simulink library "libAxisTransformations"  (R2024b)
settings: Solver=ode45  StartTime=0.0  StopTime=10.0  RelTol=1e-3  EnableMultiTasking=on
libraries: libMathOperations x14, starslibAxisTransformations x13, $bdroot x6, starslibMathOperations x2
settings Model: Creator=eheim  LastModifiedBy=gryph
settings SolverCC: AlgebraicLoopSolver=TrustRegion
settings DataIOCC: LimitDataPoints=on  SaveFormat=Array  SignalLoggingSaveFormat=ModelDataLogs  ReturnWorkspaceOutputs=off
settings OptimizationCC: ReuseModelBlockBuffer=off  ExpressionDepthLimit=2147483647  LifeSpan=inf
settings DebuggingCC: UnderspecifiedInitializationDetection=Classic  MergeDetectMultiDrivingBlocksExec=none  SolverPrmCheckMsg=warning  FcnCallInpInsideContextMsg=warning  UnconnectedInputMsg=warning  UnconnectedOutputMsg=warning  UnconnectedLineMsg=warning  StateNameClashWarn=warning  SFUnexpectedBacktrackingDiag=warning  SFNoUnconditionalDefaultTransitionDiag=warning  SFExecutionAtInitializationDiag=none  ArithmeticOperatorsInVariantConditions=warning
settings HardwareCC: ProdBitPerPointer=32  ProdBitPerSizeT=32  ProdBitPerPtrDiffT=32  ProdLargestAtomicFloat=None  ProdIntDivRoundTo=Undefined  ProdEndianess=Unspecified  ProdWordSize=32  ProdHWDeviceType=32-bit Generic
settings ModelReferenceCC: EnableRefExpFcnMdlSchedulingChecks=on  PropagateSignalLabelsOutOfModel=off
settings SFSimCC: SimUseLocalCustomCode=off  CustomCodeUndefinedFunction=UseInterfaceOnly
settings RTWCC: RTWUseLocalCustomCode=off  GPUComputeCapability=3.5  DLArmComputeVersion=19.05
settings CodeAppCC: StateflowObjectComments=on
settings GRTTargetCC: TargetLangStandard=C89/C90 (ANSI)  CombineOutputUpdateFcns=off  GRTInterface=on
settings ConfigComp: CovMetricSettings=dw  CovSaveCumulativeToWorkspaceVar=on  CovSaveSingleToWorkspaceVar=on  CovExternalEMLEnable=off  CovSFcnEnable=off

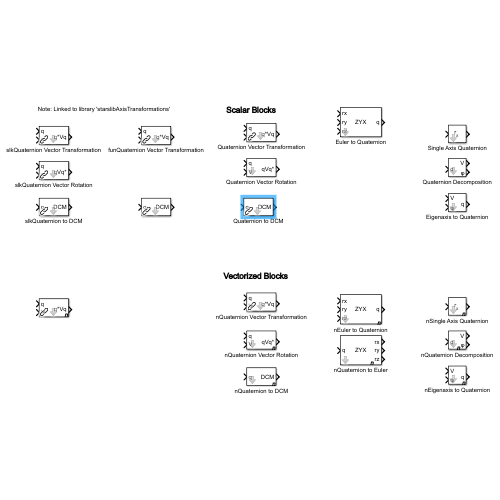
[thumbnail: Simulink's stored preview of the top-level diagram]
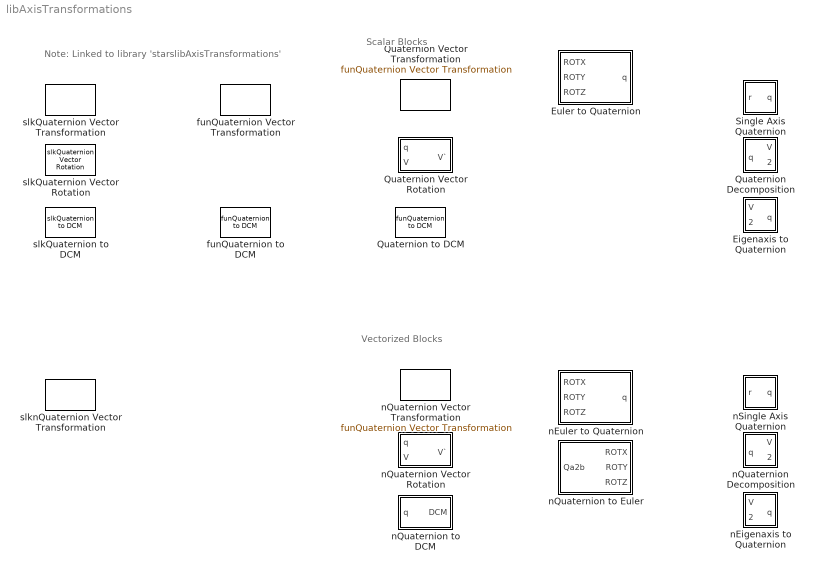
== system libAxisTransformations ==
  note: Note: Linked to library 'starslibAxisTransformations'
  note: Vectorized Blocks
  note: Scalar Blocks
  Eigenaxis to Quaternion : Subsystem  mask(Eigenaxis to Quaternion){n=0}
      mask prompts: n "Hidden variable"
      mask help: Computes quaternion from axis of rotation and angle of rotation.
      mask Display:
      | port_label('input',1,'V')
      | port_label('input',2,'\phi','texmode','on')
      | port_label('output',1,'q')
  Euler to Quaternion : Subsystem  mask(Euler to Quaternion){RotOrd=ZYX, n=0}
      mask prompts: RotOrd "Rotation Order"; n "Hidden variable"
      mask help:
      | Converts multiple Euler angle sets of
      | specified rotation order into quaternions.
      | Quat(:,K) corresponds to ROTX(1,K), ROTY(1,K),
      | and ROTZ(1,K) applied in the specified
      | order (e.g. XYZ,ZYX,...)to ultimately move from one
      | reference frame to another. ROTX, ROTY, and ROTZ
      | are inputed as row vectors with radians units.
      mask init:
      | if RotOrd==1,
      |     irt1=3;irt2=2;irt3=1;RotOrdD='ZYX';
      | elseif RotOrd==2,
      |     irt1=1;irt2=3;irt3=2;RotOrdD='XZY';
      | elseif RotOrd==3,
      |     irt1=2;irt2=1;irt3=3;RotOrdD='YXZ';
      | elseif RotOrd==4,
      |     irt1=3;irt2=1;irt3=2;RotOrdD='ZXY';    
      | elseif RotOrd==5,
      |     irt1=2;irt2=3;irt3=1;RotOrdD='YZX';    
      | elseif RotOrd==6,
      |     irt1=1;irt2=2;irt3=3;RotOrdD='XYZ';
      | end;
      mask TypeOptions RotOrd: ZYX | XZY | YXZ | ZXY | YZX | XYZ
      mask Display:
      | port_label('output',1,'q')
      | port_label('input',1,'rx')
      | port_label('input',2,'ry')
      | port_label('input',3,'rz')
      | disp(RotOrdD)
  Quaternion Decomposition : Subsystem  mask(Quaternion Decomposition){n=0}
      mask prompts: n "Hidden variable"
      mask help: Computes axis of rotation and angle of rotation of quaternion.
      mask Display:
      | port_label('input',1,'q')
      | port_label('output',1,'V')
      | port_label('output',2,'\phi','texmode','on')
  Quaternion Vector Rotation : Subsystem  mask(Quaternion Vector Rotation){n=0}
      mask prompts: n "Hidden variable"
      mask help: Produces quaternion for rotating a vector within a frame.
      mask Display:
      | port_label('input',1,'q')
      | port_label('input',2,'V')
      | port_label('output',1,'qVq*')
  Quaternion Vector Transformation : starslibAxisTransformations/funQuaternion Vector Transformation  n=0
  Quaternion to DCM : starslibAxisTransformations/funQuaternion to DCM  n=0
  Single Axis Quaternion : Subsystem  mask(Quaternion Single Axis Rotation (1-D)){RotAxis=x, n=0}
      mask prompts: RotAxis "Rotation Axis"; n "Hidden variable"
      mask help: Returns quaternion representing rotation of input angle about a selected axis. Input angle must be in radians.
      mask init:
      | switch RotAxis
      |     case 1
      |         A = [1;0;0];
      |         str = 'r_x';
      |     case 2
      |         A = [0;1;0];
      |         str = 'r_y';
      |     case 3
      |         A = [0;0;1];
      |         str = 'r_z';
      | end
      mask TypeOptions RotAxis: x | y | z
      mask Display: text(0.5,0.6,str,'texmode', 'on','HorizontalAlignment','Center','VerticalAlignment','Middle')
  funQuaternion Vector Transformation : starslibAxisTransformations/funQuaternion Vector Transformation  n=0
  funQuaternion to DCM : starslibAxisTransformations/funQuaternion to DCM  n=0
  nEigenaxis to Quaternion : Subsystem  mask(nEigenaxis to Quaternion){n=1}
      mask prompts: n "Number of Quaternions"
      mask help: Computes quaternion from axis of rotation and angle of rotation.
      mask Display:
      | port_label('input',1,'V')
      | port_label('input',2,'\phi','texmode','on')
      | port_label('output',1,'q')
      | text(1,0,'\bf\it{n}','texmode','on','HorizontalAlignment','Right','VerticalAlignment','base')
  nEuler to Quaternion : Subsystem  mask(nEuler to Quaternion){RotOrd=ZYX, n=1}
      mask prompts: RotOrd "Rotation Order"; n "Number of Quaternions"
      mask help:
      | Converts multiple Euler angle sets of
      | specified rotation order into quaternions.
      | Quat(:,K) corresponds to ROTX(1,K), ROTY(1,K),
      | and ROTZ(1,K) applied in the specified
      | order (e.g. XYZ,ZYX,...)to ultimately move from one
      | reference frame to another. ROTX, ROTY, and ROTZ
      | are inputed as row vectors with radians units.
      mask init: same as libAxisTransformations/Euler to Quaternion
      mask TypeOptions RotOrd: ZYX | XZY | YXZ | ZXY | YZX | XYZ
      mask Display:
      | port_label('output',1,'q')
      | port_label('input',1,'rx')
      | port_label('input',2,'ry')
      | port_label('input',3,'rz')
      | disp(RotOrdD)
      | text(1,0,'\bf\it{n}','texmode','on','HorizontalAlignment','Right','VerticalAlignment','base')
  nQuaternion Decomposition : Subsystem  mask(nQuaternion Decomposition){n=1}
      mask prompts: n "Number of Quaternions"
      mask help: Computes axis of rotation and angle of rotation of quaternion.
      mask Display:
      | port_label('input',1,'q')
      | port_label('output',1,'V')
      | port_label('output',2,'\phi','texmode','on')
      | text(0.5,0,'\bf\it{n}','texmode','on','HorizontalAlignment','Left','VerticalAlignment','base')
  nQuaternion Vector Rotation : Subsystem  mask(nQuaternion Vector Rotation){n=1}
      mask prompts: n "Number of Quaternions"
      mask help: Produces quaternion for rotating a vector within a frame.
      mask Display:
      | port_label('input',1,'q')
      | port_label('input',2,'V')
      | port_label('output',1,'qVq*')
      | text(1,0,'\bf\it{n}','texmode','on','HorizontalAlignment','Right','VerticalAlignment','base')
  nQuaternion Vector Transformation : starslibAxisTransformations/funQuaternion Vector Transformation  n=0
  nQuaternion to DCM : Subsystem  mask(nQuaternion to DCM){n=1}
      mask prompts: n "Number of Quaternions"
      mask help:
      | Converts n Quaternions into Direction Cosine Matrices (DCM).
      | The DCM of q(:,k) is reshape(DCM(:,k),3,3).
      mask Display:
      | port_label('input',1,'q')
      | port_label('output',1,'DCM')
      | text(1,0,'\bf\it{n}','texmode','on','HorizontalAlignment','Right','VerticalAlignment','base')
  nQuaternion to Euler : Subsystem  mask(Quaternion to Euler(4xN)){n=1, RotOrd=ZYX}
      mask prompts: n "Number of Quaternions"; RotOrd "Rotation Order"
      mask help:
      | Converts multiple quaternions (cols of input matrix)
      | into Euler angles of specified rotation order
      | (e.g. XYZ,ZYX,...).  Outputs ROTX designate rotation
      | required in x-axis, ROTY is the required rotation in the
      | y axis,and ROTZ is the required rotation in the z axis.
      | All outputs are in radians.
      mask init:
      | U1=eye(3);
      | DirCrx=[2 3; 3 1;1 2];
      | if RotOrd==1,
      |     irt1=3;irt2=2;irt3=1;RotOrdD='ZYX';
      | elseif RotOrd==2,
      |     irt1=1;irt2=3;irt3=2;RotOrdD='XZY';
      | elseif RotOrd==3,
      |     irt1=2;irt2=1;irt3=3;RotOrdD='YXZ';
      | elseif RotOrd==4,
      |     irt1=3;irt2=1;irt3=2;RotOrdD='ZXY';    
      | elseif RotOrd==5,
      |     irt1=2;irt2=3;irt3=1;RotOrdD='YZX';    
      | elseif RotOrd==6,
      |     irt1=1;irt2=2;irt3=3;RotOrdD='XYZ';
      | end;
      mask TypeOptions RotOrd: ZYX | XZY | YXZ | ZXY | YZX | XYZ
      mask Display:
      | port_label('input',1,'q')
      | port_label('output',1,'rx')
      | port_label('output',2,'ry')
      | port_label('output',3,'rz')
      | disp(RotOrdD)
      | text(0.75,0,'\bf\it{n}','texmode','on','HorizontalAlignment','Left','VerticalAlignment','base')
  nSingle Axis Quaternion : Subsystem  mask(nSingle Axis Quaternion){RotAxis=x, n=1}
      mask prompts: RotAxis "Rotation Axis"; n "Number of Angles"
      mask help: Returns quaternion(s) representing rotation(s) of input angle about a selected axis. Input angle must be in radians.
      mask init:
      | switch RotAxis
      |     case 1
      |         A = [1;0;0];
      |         str = 'r_x';
      |     case 2
      |         A = [0;1;0];
      |         str = 'r_y';
      |     case 3
      |         A = [0;0;1];
      |         str = 'r_z';
      | end
      mask TypeOptions RotAxis: x | y | z
      mask Display:
      | text(0.5,0.6,str,'texmode', 'on','HorizontalAlignment','Center','VerticalAlignment','Middle')
      | text(1,0,'\bf\it{n}','texmode','on','HorizontalAlignment','Right','VerticalAlignment','base')
  slkQuaternion Vector Rotation : starslibAxisTransformations/slkQuaternion Vector Rotation  n=0
  slkQuaternion Vector Transformation : starslibAxisTransformations/slkQuaternion Vector Transformation  n=0
  slkQuaternion to DCM : starslibAxisTransformations/slkQuaternion to DCM  n=0
  slknQuaternion Vector Transformation : starslibAxisTransformations/slknQuaternion Vector Transformation  n=1

== system libAxisTransformations/Eigenaxis to Quaternion ==
  V : Inport
  phi : Inport  Port=2
  Gain1 : Gain  Gain=0.5
  Mux : Mux  Inputs=2
  Mux1 : Mux  Inputs=3
  Normalize Vector : libMathOperations/Normalize Vector  dimnorm=rows  n=1
  Product3 : Product  RndMeth=Zero
  Quaternion Normalize : libMathOperations/Quaternion Normalize  n=0
  Trigonometric Function2 : Trigonometry  Operator=sincos
  q : Outport
  wires:
  Normalize Vector/1 -> Product3/1
  Trigonometric Function2/1 -> Mux1/2, Mux1/1, Mux1/3
  Mux1/1 -> Product3/2
  phi/1 -> Gain1/1
  Gain1/1 -> Trigonometric Function2/1
  V/1 -> Normalize Vector/1
  Product3/1 -> Mux/2
  Trigonometric Function2/2 -> Mux/1
  Mux/1 -> Quaternion Normalize/1
  Quaternion Normalize/1 -> q/1

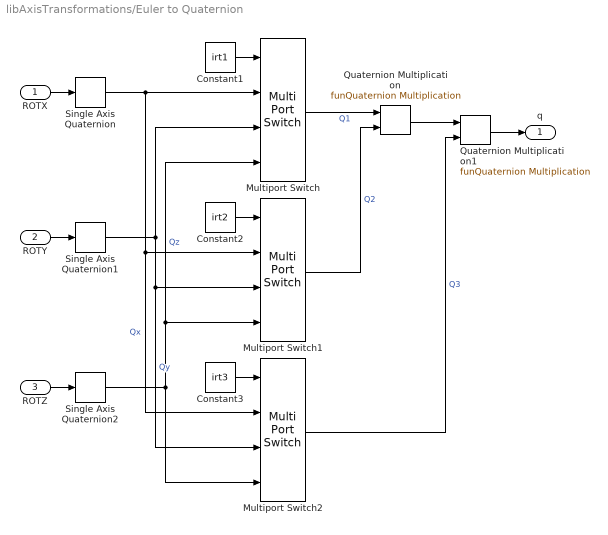
== system libAxisTransformations/Euler to Quaternion ==
  ROTX : Inport
  ROTY : Inport  Port=2
  ROTZ : Inport  Port=3
  Constant1 : Constant  Value=irt1  VectorParams1D=off
  Constant2 : Constant  Value=irt2  VectorParams1D=off
  Constant3 : Constant  Value=irt3  VectorParams1D=off
  Multiport Switch : MultiPortSwitch  SaturateOnIntegerOverflow=off  InputSameDT=off
  Multiport Switch1 : MultiPortSwitch  SaturateOnIntegerOverflow=off  InputSameDT=off
  Multiport Switch2 : MultiPortSwitch  SaturateOnIntegerOverflow=off  InputSameDT=off
  Quaternion Multiplication : starslibMathOperations/funQuaternion Multiplication  n=0
  Quaternion Multiplication1 : starslibMathOperations/funQuaternion Multiplication  n=0
  Single Axis Quaternion : $bdroot/Single Axis Quaternion  RotAxis=x  n=0
  Single Axis Quaternion1 : $bdroot/Single Axis Quaternion  RotAxis=y  n=0
  Single Axis Quaternion2 : $bdroot/Single Axis Quaternion  RotAxis=z  n=0
  q : Outport
  wires:
  Constant1/1 -> Multiport Switch/1
  Constant2/1 -> Multiport Switch1/1
  Constant3/1 -> Multiport Switch2/1
  ROTX/1 -> Single Axis Quaternion/1
  ROTZ/1 -> Single Axis Quaternion2/1
  ROTY/1 -> Single Axis Quaternion1/1
  Single Axis Quaternion/1 -> Multiport Switch/2, Multiport Switch1/2, Multiport Switch2/2  "Qx"
  Single Axis Quaternion1/1 -> Multiport Switch/3, Multiport Switch1/3, Multiport Switch2/3  "Qy"
  Single Axis Quaternion2/1 -> Multiport Switch/4, Multiport Switch1/4, Multiport Switch2/4  "Qz"
  Multiport Switch/1 -> Quaternion Multiplication/1  "Q1"
  Multiport Switch1/1 -> Quaternion Multiplication/2  "Q2"
  Quaternion Multiplication/1 -> Quaternion Multiplication1/1
  Multiport Switch2/1 -> Quaternion Multiplication1/2  "Q3"
  Quaternion Multiplication1/1 -> q/1

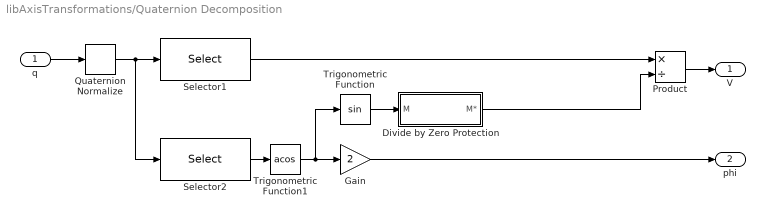
== system libAxisTransformations/Quaternion Decomposition ==
  q : Inport
  Divide by Zero Protection : Subsystem
  Gain : Gain  Gain=2
  Product : Product  Inputs=*/  RndMeth=Zero
  Quaternion Normalize : libMathOperations/Quaternion Normalize  n=0
  Selector1 : Selector  InputPortWidth=4  IndexOptions=Index vector (dialog)  Indices=[2 3 4]  OutputSizes=1
  Selector2 : Selector  InputPortWidth=4  IndexOptions=Index vector (dialog)  Indices=1  OutputSizes=1
  Trigonometric Function : Trigonometry
  Trigonometric Function1 : Trigonometry  Operator=acos
  V : Outport
  phi : Outport  Port=2
  wires:
  Divide by Zero Protection/1(M*) -> Product/2
  Trigonometric Function/1 -> Divide by Zero Protection/1(M)
  Gain/1 -> phi/1
  Trigonometric Function1/1 -> Trigonometric Function/1, Gain/1
  Selector2/1 -> Trigonometric Function1/1
  Selector1/1 -> Product/1
  Quaternion Normalize/1 -> Selector2/1, Selector1/1
  q/1 -> Quaternion Normalize/1
  Product/1 -> V/1

== system libAxisTransformations/Quaternion Vector Rotation ==
  q : Inport
  V : Inport  Port=2
  Quaternion Conjugate : libMathOperations/Quaternion Conjugate  n=0
  Subsystem6 : Subsystem  mask(Quat Mult for two special sets of quaternions){}
      mask help:
      | Quaternion multiplication of two sets of quaternions. First element assumed
      | zero of second Quaternion.  Input only last three elements
      | of second quaternion.
      mask Display:
      | disp('Quat Mult\n q0=0')
      | port_label('input',1,'p')
      | port_label('input',2,'q')
      | port_label('output',1,'p*q')
  Subsystem7 : Subsystem  mask(Quat Mult for two sets of quaternions){}
      mask help:
      | Quaternion multiplication of two sets of quaternions.  Outputs only last
      | three elements of product.
      mask Display:
      | disp('Quat Mult\n 1st Row\nRemoved')
      | port_label('input',1,'p')
      | port_label('input',2,'q')
      | port_label('output',1,'p*q')
  V` : Outport
  wires:
  Subsystem6/1(p * q) -> Subsystem7/1(p)
  q/1 -> Subsystem6/1(p), Quaternion Conjugate/1
  Subsystem7/1(p * q) -> V`/1
  V/1 -> Subsystem6/2(q)
  Quaternion Conjugate/1 -> Subsystem7/2(q)

== system libAxisTransformations/Single Axis Quaternion ==
  r : Inport
  Gain : Gain  Gain=A
  Gain3 : Gain  Gain=.5
  Mux : Mux  Inputs=2
  Trigonometric Function1 : Trigonometry  Operator=cos
  Trigonometric Function2 : Trigonometry
  q : Outport
  wires:
  Gain3/1 -> Trigonometric Function2/1, Trigonometric Function1/1
  Trigonometric Function1/1 -> Mux/1
  Gain/1 -> Mux/2
  Trigonometric Function2/1 -> Gain/1
  r/1 -> Gain3/1
  Mux/1 -> q/1

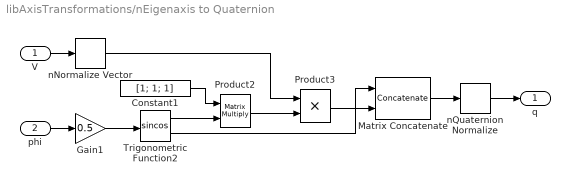
== system libAxisTransformations/nEigenaxis to Quaternion ==
  V : Inport  PortDimensions=[3,n]
  phi : Inport  Port=2  PortDimensions=[1,n]
  Constant1 : Constant  Value=[1; 1; 1]  VectorParams1D=off
  Gain1 : Gain  Gain=0.5
  Matrix Concatenate : Concatenate  Mode=Multidimensional array
  Product2 : Product  Multiplication=Matrix(*)  RndMeth=Zero
  Product3 : Product  RndMeth=Zero
  Trigonometric Function2 : Trigonometry  Operator=sincos
  nNormalize Vector : libMathOperations/nNormalize Vector  dimnorm=rows  n=[3, n]
  nQuaternion Normalize : libMathOperations/nQuaternion Normalize  n=n
  q : Outport  PortDimensions=[4,n]
  wires:
  phi/1 -> Gain1/1
  Gain1/1 -> Trigonometric Function2/1
  Constant1/1 -> Product2/1
  Trigonometric Function2/1 -> Product2/2
  Product2/1 -> Product3/2
  V/1 -> nNormalize Vector/1
  Product3/1 -> Matrix Concatenate/2
  Trigonometric Function2/2 -> Matrix Concatenate/1
  Matrix Concatenate/1 -> nQuaternion Normalize/1
  nQuaternion Normalize/1 -> q/1
  nNormalize Vector/1 -> Product3/1

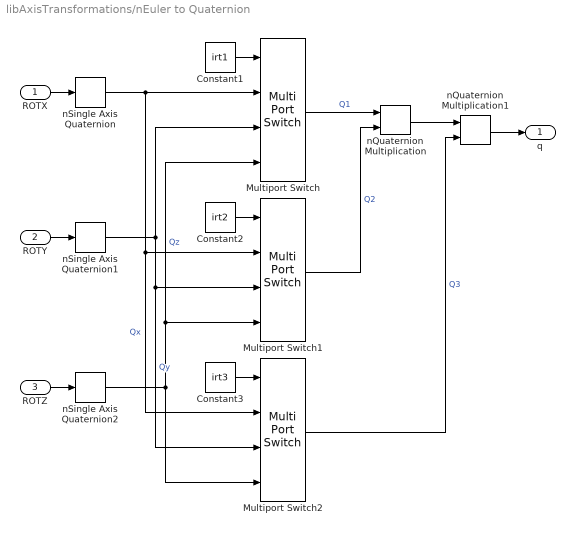
== system libAxisTransformations/nEuler to Quaternion ==
  ROTX : Inport  PortDimensions=[1,n]
  ROTY : Inport  Port=2  PortDimensions=[1,n]
  ROTZ : Inport  Port=3  PortDimensions=[1,n]
  Constant1 : Constant  Value=irt1  VectorParams1D=off
  Constant2 : Constant  Value=irt2  VectorParams1D=off
  Constant3 : Constant  Value=irt3  VectorParams1D=off
  Multiport Switch : MultiPortSwitch  SaturateOnIntegerOverflow=off  InputSameDT=off
  Multiport Switch1 : MultiPortSwitch  SaturateOnIntegerOverflow=off  InputSameDT=off
  Multiport Switch2 : MultiPortSwitch  SaturateOnIntegerOverflow=off  InputSameDT=off
  nQuaternion Multiplication : libMathOperations/nQuaternion Multiplication  n=n
  nQuaternion Multiplication1 : libMathOperations/nQuaternion Multiplication  n=n
  nSingle Axis Quaternion : $bdroot/nSingle Axis Quaternion  RotAxis=x  n=n
  nSingle Axis Quaternion1 : $bdroot/nSingle Axis Quaternion  RotAxis=y  n=n
  nSingle Axis Quaternion2 : $bdroot/nSingle Axis Quaternion  RotAxis=z  n=n
  q : Outport  PortDimensions=[4,n]
  wires:
  Constant1/1 -> Multiport Switch/1
  Constant2/1 -> Multiport Switch1/1
  Constant3/1 -> Multiport Switch2/1
  ROTX/1 -> nSingle Axis Quaternion/1
  ROTZ/1 -> nSingle Axis Quaternion2/1
  ROTY/1 -> nSingle Axis Quaternion1/1
  nSingle Axis Quaternion/1 -> Multiport Switch/2, Multiport Switch1/2, Multiport Switch2/2  "Qx"
  nSingle Axis Quaternion1/1 -> Multiport Switch/3, Multiport Switch1/3, Multiport Switch2/3  "Qy"
  nSingle Axis Quaternion2/1 -> Multiport Switch/4, Multiport Switch1/4, Multiport Switch2/4  "Qz"
  Multiport Switch/1 -> nQuaternion Multiplication/1  "Q1"
  Multiport Switch1/1 -> nQuaternion Multiplication/2  "Q2"
  nQuaternion Multiplication/1 -> nQuaternion Multiplication1/1
  Multiport Switch2/1 -> nQuaternion Multiplication1/2  "Q3"
  nQuaternion Multiplication1/1 -> q/1

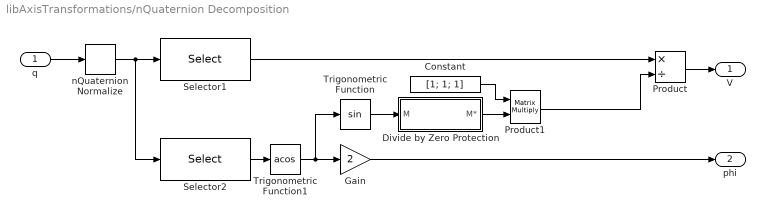
== system libAxisTransformations/nQuaternion Decomposition ==
  q : Inport  PortDimensions=[4,n]
  Constant : Constant  Value=[1; 1; 1]  VectorParams1D=off
  Divide by Zero Protection : Subsystem
  Gain : Gain  Gain=2
  Product : Product  Inputs=*/  RndMeth=Zero
  Product1 : Product  Multiplication=Matrix(*)  RndMeth=Zero
  Selector1 : Selector  NumberOfDimensions=2  InputPortWidth=3  IndexOptions=Index vector (dialog),Select all  Indices=[2 3 4],1  OutputSizes=1,1
  Selector2 : Selector  NumberOfDimensions=2  InputPortWidth=3  IndexOptions=Index vector (dialog),Select all  Indices=1,1  OutputSizes=1,1
  Trigonometric Function : Trigonometry
  Trigonometric Function1 : Trigonometry  Operator=acos
  nQuaternion Normalize : libMathOperations/nQuaternion Normalize  n=n
  V : Outport  PortDimensions=[3,n]
  phi : Outport  Port=2  PortDimensions=[1,n]
  wires:
  Divide by Zero Protection/1(M*) -> Product1/2
  Trigonometric Function/1 -> Divide by Zero Protection/1(M)
  Gain/1 -> phi/1
  Trigonometric Function1/1 -> Trigonometric Function/1, Gain/1
  Selector2/1 -> Trigonometric Function1/1
  Selector1/1 -> Product/1
  nQuaternion Normalize/1 -> Selector2/1, Selector1/1
  q/1 -> nQuaternion Normalize/1
  Product/1 -> V/1
  Product1/1 -> Product/2
  Constant/1 -> Product1/1

== system libAxisTransformations/nQuaternion Vector Rotation ==
  q : Inport  PortDimensions=[4,n]
  V : Inport  Port=2  PortDimensions=[3,n]
  Subsystem6 : Subsystem  mask(Quat Mult for two special sets of quaternions){nQuat=n}
      mask prompts: nQuat "Number of quaternions in input"
      mask help:
      | Quaternion multiplication of two sets of quaternions
      | inputted by 2 (4 x nQuat) matrices. First element assumed
      | zero of second Quaternion.  Input only last three elements
      | of second quaternion.  Used in Qtrans' first quaternion
      | multiplication
      mask Display:
      | disp('n-Quat Mult\n q0=0')
      | port_label('input',1,'p')
      | port_label('input',2,'q')
      | port_label('output',1,'p*q')
  Subsystem7 : Subsystem  mask(Quat Mult for two sets of quaternions){nQuat=n}
      mask prompts: nQuat "Number of quaternions in input"
      mask help:
      | Quaternion multiplication of two sets of quaternions
      | inputted by 2 (4 x nQuat) matrices.  Outputs only last
      | three elements of product.  Used in QTrans' second
      | multiplication
      mask Display:
      | disp('n-Quat Mult\n 1st Row\nRemoved')
      | port_label('input',1,'p')
      | port_label('input',2,'q')
      | port_label('output',1,'p*q')
  nQuaternion Conjugate : libMathOperations/nQuaternion Conjugate  n=n
  V` : Outport  PortDimensions=[3,n]
  wires:
  q/1 -> Subsystem6/1(p), nQuaternion Conjugate/1
  Subsystem6/1(p * q) -> Subsystem7/1(p)
  Subsystem7/1(p * q) -> V`/1
  V/1 -> Subsystem6/2(q)
  nQuaternion Conjugate/1 -> Subsystem7/2(q)

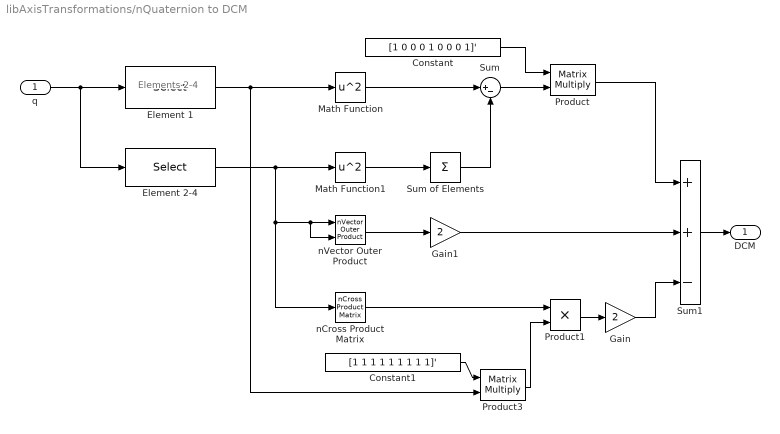
== system libAxisTransformations/nQuaternion to DCM ==
  note: Elements 2-4
  q : Inport  PortDimensions=[4,n]
  Constant : Constant  Value=[1 0 0 0 1 0 0 0 1]'  VectorParams1D=off
  Constant1 : Constant  Value=[1 1 1 1 1 1 1 1 1]'  VectorParams1D=off
  Element 1 : Selector  NumberOfDimensions=2  InputPortWidth=3  IndexOptions=Index vector (dialog),Select all  Indices=[1],1  OutputSizes=1,1
  Element 2-4 : Selector  NumberOfDimensions=2  InputPortWidth=3  IndexOptions=Index vector (dialog),Select all  Indices=[2 3 4],1  OutputSizes=1,1
  Gain : Gain  Gain=2
  Gain1 : Gain  Gain=2
  Math Function : Math  Operator=square  SignedPower=on
  Math Function1 : Math  Operator=square  SignedPower=on
  Product : Product  Multiplication=Matrix(*)  RndMeth=Zero
  Product1 : Product  RndMeth=Zero
  Product3 : Product  Multiplication=Matrix(*)  RndMeth=Zero
  Sum : Sum  Inputs=|+-
  Sum of Elements : Sum  Inputs=+  CollapseMode=Specified dimension
  Sum1 : Sum  Inputs=++-
  nCross Product Matrix : libMathOperations/nCross Product Matrix  n=n
  nVector Outer Product : libMathOperations/nVector Outer Product  n=n
  DCM : Outport  PortDimensions=[9,n]
  wires:
  Gain/1 -> Sum1/3
  Gain1/1 -> Sum1/2
  Product3/1 -> Product1/2
  Constant1/1 -> Product3/1
  nCross Product Matrix/1 -> Product1/1
  Product1/1 -> Gain/1
  Sum1/1 -> DCM/1
  Product/1 -> Sum1/1
  nVector Outer Product/1 -> Gain1/1
  Constant/1 -> Product/1
  Sum/1 -> Product/2
  Sum of Elements/1 -> Sum/2
  Math Function/1 -> Sum/1
  Math Function1/1 -> Sum of Elements/1
  Element 2-4/1 -> nVector Outer Product/1, nVector Outer Product/2, nCross Product Matrix/1, Math Function1/1
  Element 1/1 -> Product3/2, Math Function/1
  q/1 -> Element 1/1, Element 2-4/1

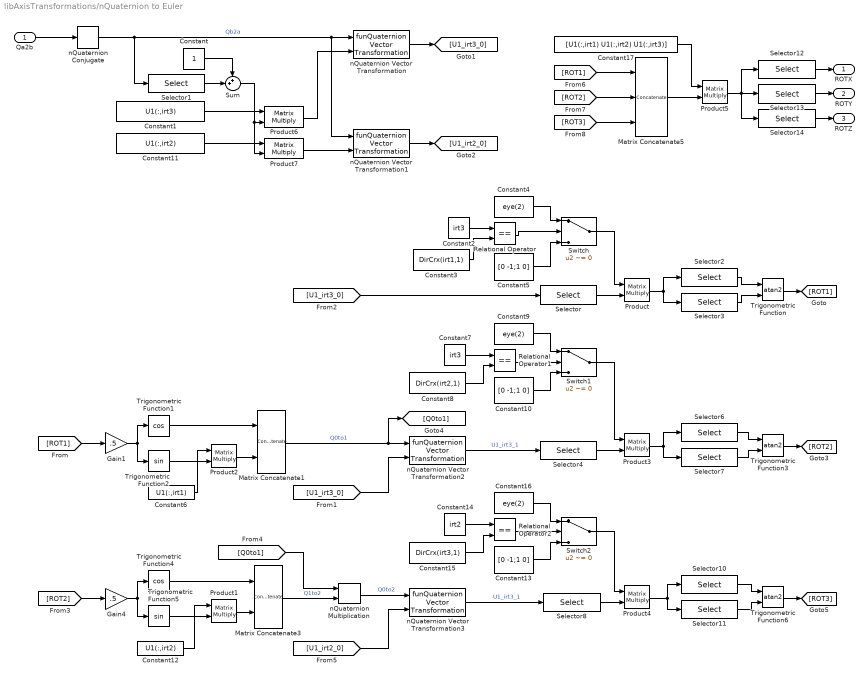
== system libAxisTransformations/nQuaternion to Euler ==
  Qa2b : Inport  PortDimensions=[4,n]
  Constant : Constant
  Constant1 : Constant  Value=U1(:,irt3)  VectorParams1D=off
  Constant10 : Constant  Value=[0 -1;1 0]  VectorParams1D=off
  Constant11 : Constant  Value=U1(:,irt2)  VectorParams1D=off
  Constant12 : Constant  Value=U1(:,irt2)  VectorParams1D=off
  Constant13 : Constant  Value=[0 -1;1 0]  VectorParams1D=off
  Constant14 : Constant  Value=irt2  VectorParams1D=off
  Constant15 : Constant  Value=DirCrx(irt3,1)  VectorParams1D=off
  Constant16 : Constant  Value=eye(2)  VectorParams1D=off
  Constant17 : Constant  Value=[U1(:,irt1) U1(:,irt2) U1(:,irt3)]  VectorParams1D=off
  Constant2 : Constant  Value=irt3  VectorParams1D=off
  Constant3 : Constant  Value=DirCrx(irt1,1)  VectorParams1D=off
  Constant4 : Constant  Value=eye(2)  VectorParams1D=off
  Constant5 : Constant  Value=[0 -1;1 0]  VectorParams1D=off
  Constant6 : Constant  Value=U1(:,irt1)  VectorParams1D=off
  Constant7 : Constant  Value=irt3  VectorParams1D=off
  Constant8 : Constant  Value=DirCrx(irt2,1)  VectorParams1D=off
  Constant9 : Constant  Value=eye(2)  VectorParams1D=off
  Gain1 : Gain  Gain=.5
  Gain4 : Gain  Gain=.5
  Matrix Concatenate1 : Concatenate  Mode=Multidimensional array
  Matrix Concatenate3 : Concatenate  Mode=Multidimensional array
  Matrix Concatenate5 : Concatenate  NumInputs=3  Mode=Multidimensional array
  Product{,1..7} (8 alike) : Product  Multiplication=Matrix(*)  RndMeth=Zero
  Relational Operator : RelationalOperator  Operator===  OutDataTypeStr=boolean  ZeroCross=off  InputSameDT=off
  Relational Operator1 : RelationalOperator  Operator===  OutDataTypeStr=boolean  ZeroCross=off  InputSameDT=off
  Relational Operator2 : RelationalOperator  Operator===  OutDataTypeStr=boolean  ZeroCross=off  InputSameDT=off
  Selector : Selector  NumberOfDimensions=2  InputPortWidth=3  IndexOptions=Index vector (dialog),Select all  Indices=[DirCrx(irt1,2) DirCrx(irt1,1)],1  OutputSizes=1,1
  Selector{1..2,6,10,12} (5 alike) : Selector  NumberOfDimensions=2  InputPortWidth=3  IndexOptions=Index vector (dialog),Select all  Indices=1,1  OutputSizes=1,1
  Selector{3,7,11,13} (4 alike) : Selector  NumberOfDimensions=2  InputPortWidth=3  IndexOptions=Index vector (dialog),Select all  Indices=2,1  OutputSizes=1,1
  Selector14 : Selector  NumberOfDimensions=2  InputPortWidth=3  IndexOptions=Index vector (dialog),Select all  Indices=3,1  OutputSizes=1,1
  Selector4 : Selector  NumberOfDimensions=2  InputPortWidth=3  IndexOptions=Index vector (dialog),Select all  Indices=[DirCrx(irt2,2) DirCrx(irt2,1)],1  OutputSizes=1,1
  Selector8 : Selector  NumberOfDimensions=2  InputPortWidth=3  IndexOptions=Index vector (dialog),Select all  Indices=[DirCrx(irt3,2) DirCrx(irt3,1)],1  OutputSizes=1,1
  Sum : Sum  Inputs=++|
  Switch : Switch  Criteria=u2 ~= 0  ZeroCross=off  SaturateOnIntegerOverflow=off  InputSameDT=off
  Switch1 : Switch  Criteria=u2 ~= 0  ZeroCross=off  SaturateOnIntegerOverflow=off  InputSameDT=off
  Switch2 : Switch  Criteria=u2 ~= 0  ZeroCross=off  SaturateOnIntegerOverflow=off  InputSameDT=off
  Trigonometric Function : Trigonometry  Operator=atan2
  Trigonometric Function1 : Trigonometry  Operator=cos
  Trigonometric Function2 : Trigonometry
  Trigonometric Function3 : Trigonometry  Operator=atan2
  Trigonometric Function4 : Trigonometry  Operator=cos
  Trigonometric Function5 : Trigonometry
  Trigonometric Function6 : Trigonometry  Operator=atan2
  nQuaternion Conjugate : libMathOperations/nQuaternion Conjugate  n=n
  nQuaternion Multiplication : libMathOperations/nQuaternion Multiplication  n=n
  nQuaternion Vector Transformation{,1..3} (4 alike) : starslibAxisTransformations/funQuaternion Vector Transformation  n=n
  ROTX : Outport  PortDimensions=[1,n]
  ROTY : Outport  Port=2  PortDimensions=[1,n]
  ROTZ : Outport  Port=3  PortDimensions=[1,n]
  wires:
  nQuaternion Conjugate/1 -> nQuaternion Vector Transformation/1, nQuaternion Vector Transformation1/1, Selector1/1  "Qb2a"
  nQuaternion Vector Transformation/1 -> [U1_irt3_0]
  Constant2/1 -> Relational Operator/1
  Constant3/1 -> Relational Operator/2
  Relational Operator/1 -> Switch/2
  Selector/1 -> Product/2
  Constant4/1 -> Switch/1
  Constant5/1 -> Switch/3
  Switch/1 -> Product/1
  Product/1 -> Selector2/1, Selector3/1
  Selector2/1 -> Trigonometric Function/1
  Selector3/1 -> Trigonometric Function/2
  Trigonometric Function/1 -> [ROT1]
  Gain1/1 -> Trigonometric Function1/1, Trigonometric Function2/1
  Constant6/1 -> Product2/1
  Trigonometric Function2/1 -> Product2/2
  Product2/1 -> Matrix Concatenate1/2
  Trigonometric Function1/1 -> Matrix Concatenate1/1
  Matrix Concatenate1/1 -> [Q0to1], nQuaternion Vector Transformation2/1  "Q0to1"
  Constant7/1 -> Relational Operator1/1
  Constant8/1 -> Relational Operator1/2
  Relational Operator1/1 -> Switch1/2
  Constant9/1 -> Switch1/1
  Constant10/1 -> Switch1/3
  nQuaternion Vector Transformation2/1 -> Selector4/1  "U1_irt3_1"
  Selector4/1 -> Product3/2
  Product3/1 -> Selector6/1, Selector7/1
  Selector6/1 -> Trigonometric Function3/1
  Selector7/1 -> Trigonometric Function3/2
  [ROT1] -> Gain1/1
  [U1_irt3_0] -> nQuaternion Vector Transformation2/2
  [U1_irt3_0] -> Selector/1
  nQuaternion Vector Transformation1/1 -> [U1_irt2_0]
  Trigonometric Function3/1 -> [ROT2]
  Gain4/1 -> Trigonometric Function4/1, Trigonometric Function5/1
  Constant12/1 -> Product1/1
  Trigonometric Function5/1 -> Product1/2
  Product1/1 -> Matrix Concatenate3/2
  Trigonometric Function4/1 -> Matrix Concatenate3/1
  [ROT2] -> Gain4/1
  Matrix Concatenate3/1 -> nQuaternion Multiplication/2  "Q1to2"
  [Q0to1] -> nQuaternion Multiplication/1
  nQuaternion Multiplication/1 -> nQuaternion Vector Transformation3/1  "Q0to2"
  [U1_irt2_0] -> nQuaternion Vector Transformation3/2
  Constant14/1 -> Relational Operator2/1
  Constant15/1 -> Relational Operator2/2
  Relational Operator2/1 -> Switch2/2
  Constant16/1 -> Switch2/1
  Constant13/1 -> Switch2/3
  nQuaternion Vector Transformation3/1 -> Selector8/1  "U1_irt3_1"
  Selector8/1 -> Product4/2
  Switch2/1 -> Product4/1
  Product4/1 -> Selector10/1, Selector11/1
  Selector10/1 -> Trigonometric Function6/1
  Selector11/1 -> Trigonometric Function6/2
  Trigonometric Function6/1 -> [ROT3]
  [ROT1] -> Matrix Concatenate5/1
  [ROT2] -> Matrix Concatenate5/2
  [ROT3] -> Matrix Concatenate5/3
  Matrix Concatenate5/1 -> Product5/2
  Constant17/1 -> Product5/1
  Product5/1 -> Selector12/1, Selector13/1, Selector14/1
  Qa2b/1 -> nQuaternion Conjugate/1
  Selector12/1 -> ROTX/1
  Selector13/1 -> ROTY/1
  Selector14/1 -> ROTZ/1
  Switch1/1 -> Product3/1
  Constant/1 -> Sum/1
  Selector1/1 -> Sum/2
  Product6/1 -> nQuaternion Vector Transformation/2
  Product7/1 -> nQuaternion Vector Transformation1/2
  Sum/1 -> Product6/2, Product7/2
  Constant1/1 -> Product6/1
  Constant11/1 -> Product7/1

== system libAxisTransformations/nSingle Axis Quaternion ==
  r : Inport  PortDimensions=[1,n]
  Constant6 : Constant  Value=A  VectorParams1D=off
  Gain3 : Gain  Gain=.5
  Matrix Concatenate1 : Concatenate  Mode=Multidimensional array
  Product2 : Product  Multiplication=Matrix(*)  RndMeth=Zero
  Trigonometric Function1 : Trigonometry  Operator=cos
  Trigonometric Function2 : Trigonometry
  q : Outport  PortDimensions=[4,n]
  wires:
  Trigonometric Function1/1 -> Matrix Concatenate1/1
  Product2/1 -> Matrix Concatenate1/2
  Trigonometric Function2/1 -> Product2/2
  Constant6/1 -> Product2/1
  Gain3/1 -> Trigonometric Function2/1, Trigonometric Function1/1
  r/1 -> Gain3/1
  Matrix Concatenate1/1 -> q/1

== system libAxisTransformations/Quaternion Decomposition/Divide by Zero Protection ==
  note: Replace magnitudes equal to 0 by 1
  M : Inport
  Constant : Constant
  Switch : Switch  Criteria=u2 ~= 0  SaturateOnIntegerOverflow=off  InputSameDT=off
  M* : Outport
  wires:
  M/1 -> Switch/1, Switch/2
  Constant/1 -> Switch/3
  Switch/1 -> M*/1

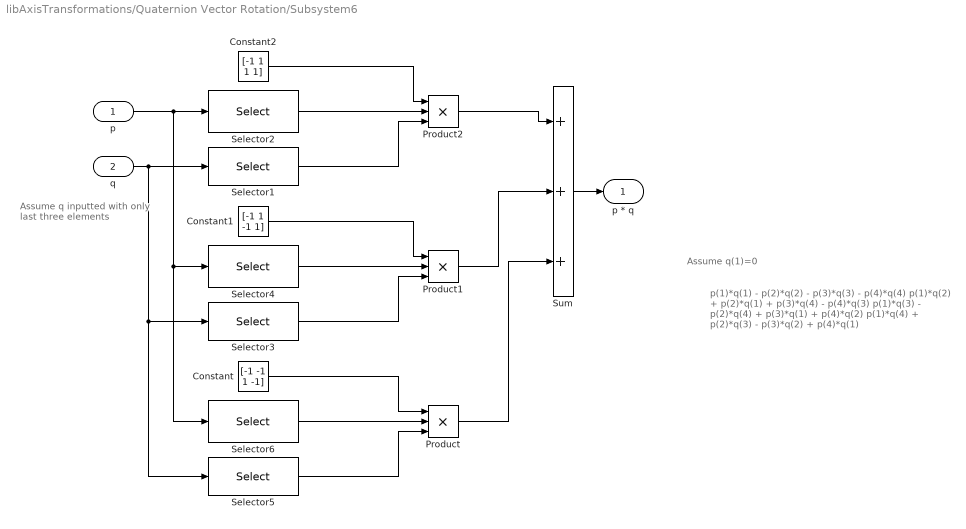
== system libAxisTransformations/Quaternion Vector Rotation/Subsystem6 ==
  note: p(1)*q(1) - p(2)*q(2) - p(3)*q(3) - p(4)*q(4)
      |
      | p(1)*q(2) + p(2)*q(1) + p(3)*q(4) - p(4)*q(3)
      |
      | p(1)*q(3) - p(2)*q(4) + p(3)*q(1) + p(4)*q(2)
      |
      | p(1)*q(4) + p(2)*q(3) - p(3)*q(2) + p(4)*q(1)
  note: Assume q(1)=0
  note: Assume q
      | inputted with only
      | last three elements
  p : Inport
  q : Inport  Port=2
  Constant : Constant  Value=[-1 -1 1 -1]
  Constant1 : Constant  Value=[-1 1 -1 1]
  Constant2 : Constant  Value=[-1 1 1 1]
  Product : Product  Inputs=3  RndMeth=Zero
  Product1 : Product  Inputs=3  RndMeth=Zero
  Product2 : Product  Inputs=3  RndMeth=Zero
  Selector1 : Selector  InputPortWidth=3  IndexOptions=Index vector (dialog)  Indices=[1 1 2 3]  OutputSizes=1
  Selector2 : Selector  InputPortWidth=4  IndexOptions=Index vector (dialog)  Indices=[2 1 1 1]  OutputSizes=1
  Selector3 : Selector  InputPortWidth=3  IndexOptions=Index vector (dialog)  Indices=[2 3 3 2]  OutputSizes=1
  Selector4 : Selector  InputPortWidth=4  IndexOptions=Index vector (dialog)  Indices=[3 3 2 2]  OutputSizes=1
  Selector5 : Selector  InputPortWidth=3  IndexOptions=Index vector (dialog)  Indices=[3 2 1 1]  OutputSizes=1
  Selector6 : Selector  InputPortWidth=4  IndexOptions=Index vector (dialog)  Indices=[4 4 4 3]  OutputSizes=1
  Sum : Sum  Inputs=+++
  p * q : Outport
  wires:
  Constant1/1 -> Product1/1
  Constant2/1 -> Product2/1
  Constant/1 -> Product/1
  Selector4/1 -> Product1/2
  Selector6/1 -> Product/2
  Selector1/1 -> Product2/3
  Selector3/1 -> Product1/3
  Selector5/1 -> Product/3
  Product2/1 -> Sum/1
  Product1/1 -> Sum/2
  Product/1 -> Sum/3
  p/1 -> Selector2/1, Selector4/1, Selector6/1
  q/1 -> Selector1/1, Selector3/1, Selector5/1
  Sum/1 -> p * q/1
  Selector2/1 -> Product2/2

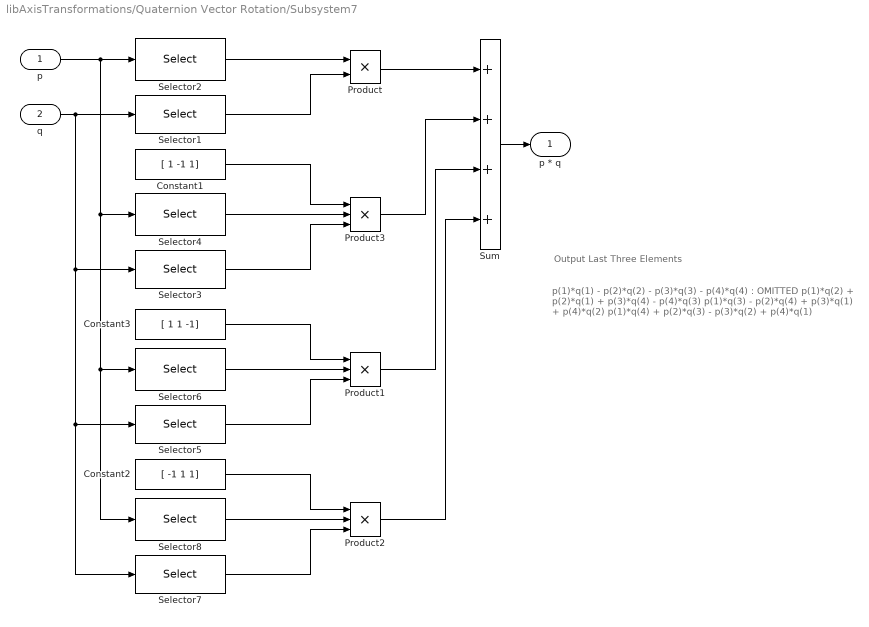
== system libAxisTransformations/Quaternion Vector Rotation/Subsystem7 ==
  note: Output Last Three Elements
  note: p(1)*q(1) - p(2)*q(2) - p(3)*q(3) - p(4)*q(4) :  OMITTED
      |
      | p(1)*q(2) + p(2)*q(1) + p(3)*q(4) - p(4)*q(3)
      |
      | p(1)*q(3) - p(2)*q(4) + p(3)*q(1) + p(4)*q(2)
      |
      | p(1)*q(4) + p(2)*q(3) - p(3)*q(2) + p(4)*q(1)
  p : Inport
  q : Inport  Port=2
  Constant1 : Constant  Value=[ 1 -1 1]
  Constant2 : Constant  Value=[ -1 1 1]
  Constant3 : Constant  Value=[ 1 1 -1]
  Product : Product  RndMeth=Zero
  Product1 : Product  Inputs=3  RndMeth=Zero
  Product2 : Product  Inputs=3  RndMeth=Zero
  Product3 : Product  Inputs=3  RndMeth=Zero
  Selector1 : Selector  InputPortWidth=4  IndexOptions=Index vector (dialog)  Indices=[ 2 3 4]  OutputSizes=1
  Selector2 : Selector  InputPortWidth=4  IndexOptions=Index vector (dialog)  Indices=[ 1 1 1]  OutputSizes=1
  Selector3 : Selector  InputPortWidth=4  IndexOptions=Index vector (dialog)  Indices=[ 1 4 3]  OutputSizes=1
  Selector4 : Selector  InputPortWidth=4  IndexOptions=Index vector (dialog)  Indices=[ 2 2 2]  OutputSizes=1
  Selector5 : Selector  InputPortWidth=4  IndexOptions=Index vector (dialog)  Indices=[ 4 1 2]  OutputSizes=1
  Selector6 : Selector  InputPortWidth=4  IndexOptions=Index vector (dialog)  Indices=[ 3 3 3]  OutputSizes=1
  Selector7 : Selector  InputPortWidth=4  IndexOptions=Index vector (dialog)  Indices=[ 3 2 1]  OutputSizes=1
  Selector8 : Selector  InputPortWidth=4  IndexOptions=Index vector (dialog)  Indices=[4 4 4]  OutputSizes=1
  Sum : Sum  Inputs=++++
  p * q : Outport
  wires:
  Selector5/1 -> Product1/3
  Selector6/1 -> Product1/2
  Constant3/1 -> Product1/1
  Selector7/1 -> Product2/3
  Selector8/1 -> Product2/2
  Constant2/1 -> Product2/1
  Selector3/1 -> Product3/3
  Selector4/1 -> Product3/2
  Constant1/1 -> Product3/1
  Selector1/1 -> Product/2
  Selector2/1 -> Product/1
  Sum/1 -> p * q/1
  q/1 -> Selector7/1, Selector5/1, Selector3/1, Selector1/1
  p/1 -> Selector8/1, Selector6/1, Selector4/1, Selector2/1
  Product2/1 -> Sum/4
  Product1/1 -> Sum/3
  Product3/1 -> Sum/2
  Product/1 -> Sum/1

== system libAxisTransformations/nQuaternion Decomposition/Divide by Zero Protection ==
  note: Replace magnitudes equal to 0 by 1
  M : Inport
  Constant : Constant
  Switch : Switch  Criteria=u2 ~= 0  ZeroCross=off  SaturateOnIntegerOverflow=off  InputSameDT=off
  M* : Outport
  wires:
  M/1 -> Switch/1, Switch/2
  Constant/1 -> Switch/3
  Switch/1 -> M*/1

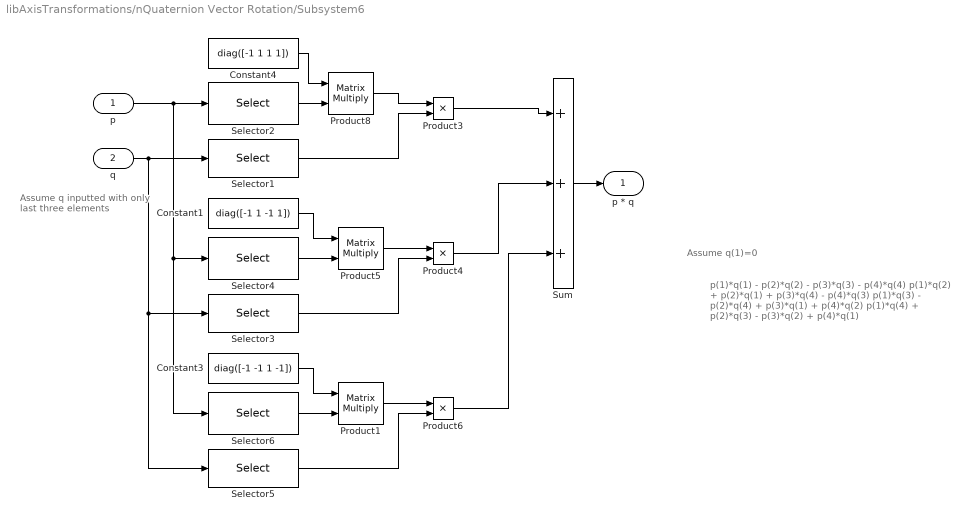
== system libAxisTransformations/nQuaternion Vector Rotation/Subsystem6 ==
  note: Assume q
      | inputted with only
      | last three elements
  note: Assume q(1)=0
  note: p(1)*q(1) - p(2)*q(2) - p(3)*q(3) - p(4)*q(4)
      |
      | p(1)*q(2) + p(2)*q(1) + p(3)*q(4) - p(4)*q(3)
      |
      | p(1)*q(3) - p(2)*q(4) + p(3)*q(1) + p(4)*q(2)
      |
      | p(1)*q(4) + p(2)*q(3) - p(3)*q(2) + p(4)*q(1)
  p : Inport  PortDimensions=[4,nQuat]
  q : Inport  Port=2  PortDimensions=[3,nQuat]
  Constant1 : Constant  Value=diag([-1 1 -1 1])  VectorParams1D=off
  Constant3 : Constant  Value=diag([-1 -1 1 -1])  VectorParams1D=off
  Constant4 : Constant  Value=diag([-1 1 1 1])  VectorParams1D=off
  Product1 : Product  Multiplication=Matrix(*)  RndMeth=Zero
  Product3 : Product  RndMeth=Zero
  Product4 : Product  RndMeth=Zero
  Product5 : Product  Multiplication=Matrix(*)  RndMeth=Zero
  Product6 : Product  RndMeth=Zero
  Product8 : Product  Multiplication=Matrix(*)  RndMeth=Zero
  Selector1 : Selector  NumberOfDimensions=2  InputPortWidth=3  IndexOptions=Index vector (dialog),Select all  Indices=[1 1 2 3],1  OutputSizes=1,1
  Selector2 : Selector  NumberOfDimensions=2  InputPortWidth=3  IndexOptions=Index vector (dialog),Select all  Indices=[2 1 1 1],1  OutputSizes=1,1
  Selector3 : Selector  NumberOfDimensions=2  InputPortWidth=3  IndexOptions=Index vector (dialog),Select all  Indices=[2 3 3 2],1  OutputSizes=1,1
  Selector4 : Selector  NumberOfDimensions=2  InputPortWidth=3  IndexOptions=Index vector (dialog),Select all  Indices=[3 3 2 2],1  OutputSizes=1,1
  Selector5 : Selector  NumberOfDimensions=2  InputPortWidth=3  IndexOptions=Index vector (dialog),Select all  Indices=[3 2 1 1],1  OutputSizes=1,1
  Selector6 : Selector  NumberOfDimensions=2  InputPortWidth=3  IndexOptions=Index vector (dialog),Select all  Indices=[4 4 4 3],1  OutputSizes=1,1
  Sum : Sum  Inputs=+++
  p * q : Outport  PortDimensions=[4,nQuat]
  wires:
  Constant4/1 -> Product8/1
  Product8/1 -> Product3/1
  Selector2/1 -> Product8/2
  Sum/1 -> p * q/1
  q/1 -> Selector5/1, Selector3/1, Selector1/1
  p/1 -> Selector6/1, Selector4/1, Selector2/1
  Product6/1 -> Sum/3
  Product4/1 -> Sum/2
  Product3/1 -> Sum/1
  Selector5/1 -> Product6/2
  Product1/1 -> Product6/1
  Selector3/1 -> Product4/2
  Product5/1 -> Product4/1
  Selector1/1 -> Product3/2
  Constant3/1 -> Product1/1
  Selector6/1 -> Product1/2
  Constant1/1 -> Product5/1
  Selector4/1 -> Product5/2

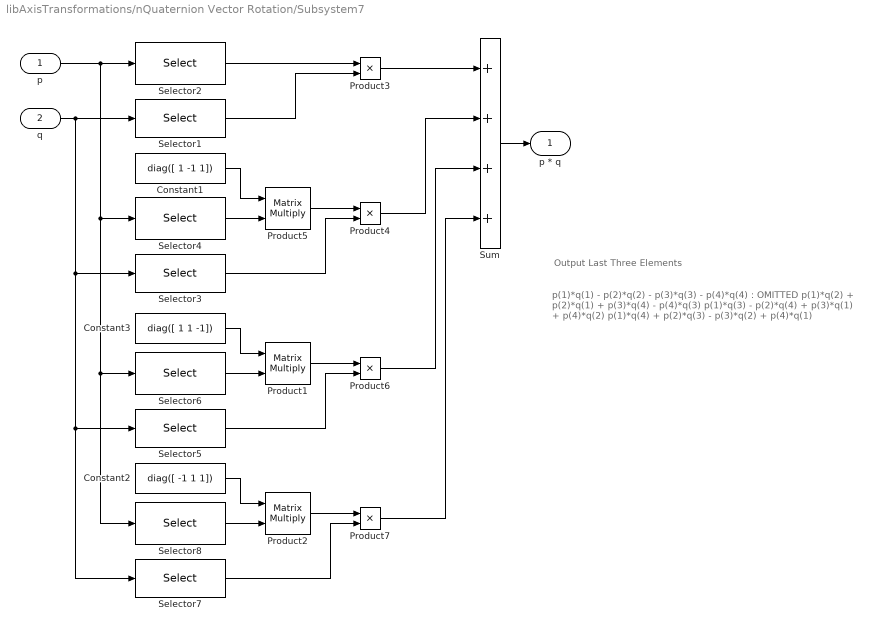
== system libAxisTransformations/nQuaternion Vector Rotation/Subsystem7 ==
  note: Output Last Three Elements
  note: p(1)*q(1) - p(2)*q(2) - p(3)*q(3) - p(4)*q(4) :  OMITTED
      |
      | p(1)*q(2) + p(2)*q(1) + p(3)*q(4) - p(4)*q(3)
      |
      | p(1)*q(3) - p(2)*q(4) + p(3)*q(1) + p(4)*q(2)
      |
      | p(1)*q(4) + p(2)*q(3) - p(3)*q(2) + p(4)*q(1)
  p : Inport  PortDimensions=[4,nQuat]
  q : Inport  Port=2  PortDimensions=[4,nQuat]
  Constant1 : Constant  Value=diag([ 1 -1 1])  VectorParams1D=off
  Constant2 : Constant  Value=diag([ -1 1 1])  VectorParams1D=off
  Constant3 : Constant  Value=diag([ 1 1 -1])  VectorParams1D=off
  Product1 : Product  Multiplication=Matrix(*)  RndMeth=Zero
  Product2 : Product  Multiplication=Matrix(*)  RndMeth=Zero
  Product{3..4,6..7} (4 alike) : Product  RndMeth=Zero
  Product5 : Product  Multiplication=Matrix(*)  RndMeth=Zero
  Selector1 : Selector  NumberOfDimensions=2  InputPortWidth=3  IndexOptions=Index vector (dialog),Select all  Indices=[ 2 3 4],1  OutputSizes=1,1
  Selector2 : Selector  NumberOfDimensions=2  InputPortWidth=3  IndexOptions=Index vector (dialog),Select all  Indices=[ 1 1 1],1  OutputSizes=1,1
  Selector3 : Selector  NumberOfDimensions=2  InputPortWidth=3  IndexOptions=Index vector (dialog),Select all  Indices=[ 1 4 3],1  OutputSizes=1,1
  Selector4 : Selector  NumberOfDimensions=2  InputPortWidth=3  IndexOptions=Index vector (dialog),Select all  Indices=[ 2 2 2],1  OutputSizes=1,1
  Selector5 : Selector  NumberOfDimensions=2  InputPortWidth=3  IndexOptions=Index vector (dialog),Select all  Indices=[ 4 1 2],1  OutputSizes=1,1
  Selector6 : Selector  NumberOfDimensions=2  InputPortWidth=3  IndexOptions=Index vector (dialog),Select all  Indices=[ 3 3 3],1  OutputSizes=1,1
  Selector7 : Selector  NumberOfDimensions=2  InputPortWidth=3  IndexOptions=Index vector (dialog),Select all  Indices=[ 3 2 1],1  OutputSizes=1,1
  Selector8 : Selector  NumberOfDimensions=2  InputPortWidth=3  IndexOptions=Index vector (dialog),Select all  Indices=[4 4 4],1  OutputSizes=1,1
  Sum : Sum  Inputs=++++
  p * q : Outport  PortDimensions=[3,nQuat]
  wires:
  Sum/1 -> p * q/1
  q/1 -> Selector7/1, Selector5/1, Selector3/1, Selector1/1
  p/1 -> Selector8/1, Selector6/1, Selector4/1, Selector2/1
  Product7/1 -> Sum/4
  Product6/1 -> Sum/3
  Product4/1 -> Sum/2
  Product3/1 -> Sum/1
  Selector7/1 -> Product7/2
  Product2/1 -> Product7/1
  Selector5/1 -> Product6/2
  Product1/1 -> Product6/1
  Selector3/1 -> Product4/2
  Product5/1 -> Product4/1
  Selector1/1 -> Product3/2
  Selector2/1 -> Product3/1
  Constant2/1 -> Product2/1
  Selector8/1 -> Product2/2
  Constant3/1 -> Product1/1
  Selector6/1 -> Product1/2
  Constant1/1 -> Product5/1
  Selector4/1 -> Product5/2
